simulink model "Copy_of_modelo_completo_sin_joystick"  (R2021a)
settings: Solver=FixedStepAuto  StartTime=0.0  StopTime=inf  FixedStep=0.001  MaxStep=1e-4  RelTol=1e-3
undefined symbols (not defined in the file): bah, bat, bcx, bcy, beqhd, beqt, bw, C_HEIGHT, cols_centers, cols_height, cont_mass, ddxmax, ddxmin, ddymax, ddymin, g, Kcy, Ksah, Ksat, Ksiah, Ksiat, Kw, lh0, Meqh, Meqt, mt, Rd, rt, rth, Rw, sigbuilder_block, sp_mass, VH_MAX, VT_MAX, w_mt_h, w_mt_i, xmax, xt0, ymax, yt0
libraries: simulink x1
(part 2 of 2)

== stateflow chart Copy_of_modelo_completo_sin_joystick/Control Level 1 - Global Supervisor Control1 ==
  state LEVEL1
    entry:
    heights = cols_height;
    centers = cols_centers;
    p0=[0,0];p1=[0,0];p2=[0,0];p3=[0,0];p4=[0,0];p5=[0,0];p6=[0,0];p7=[0,0];p12=[0,0];p23=[0,0];p34=[0,0];p45=[0,0];p56=[0,0];
    [p0,p1,p2,p3,p4,p5,p6,p7,p12,p23,p34,p45,p56] = generate_trajectory(ml,VH_MAX,VT_MAX,heights,centers,single_cycle,double_cycle);
    state MOVEMENT [parallel]
      settings: executionOrder=2
      state AUTOMATIC
        state TO_SHIP
          state HOISTING_ONLY
            state INIT
            state UP
              dxt = 0;
              dlh = -VH_MAX;
            state DOWN
              dxt = 0;
              dlh = VH_MAX;
            (default) -> LEVEL1.MOVEMENT.AUTOMATIC.TO_SHIP.HOISTING_ONLY.INIT
            LEVEL1.MOVEMENT.AUTOMATIC.TO_SHIP.HOISTING_ONLY.INIT -> LEVEL1.MOVEMENT.AUTOMATIC.TO_SHIP.HOISTING_ONLY.DOWN [order 1] : [current_stage==5 && prev_stage==4]
            LEVEL1.MOVEMENT.AUTOMATIC.TO_SHIP.HOISTING_ONLY.INIT -> LEVEL1.MOVEMENT.AUTOMATIC.TO_SHIP.HOISTING_ONLY.UP [order 2] : [current_stage==1&& prev_stage==0]
          state INIT
          state HOISTING_AND_TROLLEY
            state UP
              dxt = VT_MAX;
              dlh = -VH_MAX;
            state DOWN
              dxt = VT_MAX;
              dlh = VH_MAX;
            state INIT
            (default) -> LEVEL1.MOVEMENT.AUTOMATIC.TO_SHIP.HOISTING_AND_TROLLEY.INIT
            LEVEL1.MOVEMENT.AUTOMATIC.TO_SHIP.HOISTING_AND_TROLLEY.INIT -> LEVEL1.MOVEMENT.AUTOMATIC.TO_SHIP.HOISTING_AND_TROLLEY.UP [order 1] : [current_stage == 2 && prev_stage == 1]
            LEVEL1.MOVEMENT.AUTOMATIC.TO_SHIP.HOISTING_AND_TROLLEY.INIT -> LEVEL1.MOVEMENT.AUTOMATIC.TO_SHIP.HOISTING_AND_TROLLEY.DOWN [order 2] : [current_stage== 4 && prev_stage == 3]
          state TROLLEY_ONLY
            dxt = VT_MAX
            dlh = 0;
          (default) -> LEVEL1.MOVEMENT.AUTOMATIC.TO_SHIP.INIT
          LEVEL1.MOVEMENT.AUTOMATIC.TO_SHIP.INIT -> LEVEL1.MOVEMENT.AUTOMATIC.TO_SHIP.HOISTING_ONLY
          LEVEL1.MOVEMENT.AUTOMATIC.TO_SHIP.HOISTING_ONLY -> LEVEL1.MOVEMENT.AUTOMATIC.TO_SHIP.HOISTING_AND_TROLLEY : [current_stage==2 && prev_stage==1]
          LEVEL1.MOVEMENT.AUTOMATIC.TO_SHIP.HOISTING_AND_TROLLEY -> LEVEL1.MOVEMENT.AUTOMATIC.TO_SHIP.HOISTING_ONLY [order 2] : [current_stage == 5 && prev_stage == 4]
          LEVEL1.MOVEMENT.AUTOMATIC.TO_SHIP.HOISTING_AND_TROLLEY -> LEVEL1.MOVEMENT.AUTOMATIC.TO_SHIP.TROLLEY_ONLY [order 1] : [current_stage==3 && prev_stage==2]
          LEVEL1.MOVEMENT.AUTOMATIC.TO_SHIP.TROLLEY_ONLY -> LEVEL1.MOVEMENT.AUTOMATIC.TO_SHIP.HOISTING_AND_TROLLEY : [current_stage == 4 && prev_stage == 3]
        state INIT
        state TO_DOCK
          state HOISTING_ONLY
            state UP
              dxt = 0;
              dlh = -VH_MAX;
            state INIT
            state DOWN
              dxt = 0;
              dlh = VH_MAX;
            (default) -> LEVEL1.MOVEMENT.AUTOMATIC.TO_DOCK.HOISTING_ONLY.INIT
            LEVEL1.MOVEMENT.AUTOMATIC.TO_DOCK.HOISTING_ONLY.INIT -> LEVEL1.MOVEMENT.AUTOMATIC.TO_DOCK.HOISTING_ONLY.UP [order 1] : [current_stage == 5 && prev_stage == 6]
            LEVEL1.MOVEMENT.AUTOMATIC.TO_DOCK.HOISTING_ONLY.INIT -> LEVEL1.MOVEMENT.AUTOMATIC.TO_DOCK.HOISTING_ONLY.DOWN [order 2] : [current_stage == 1&& prev_stage == 2]
          state INIT
          state HOISTING_AND_TROLLEY
            state UP
              dxt = -VT_MAX;
              dlh = -VH_MAX;
            state INIT
            state DOWN
              dxt = -VT_MAX;
              dlh = VH_MAX;
            (default) -> LEVEL1.MOVEMENT.AUTOMATIC.TO_DOCK.HOISTING_AND_TROLLEY.INIT
            LEVEL1.MOVEMENT.AUTOMATIC.TO_DOCK.HOISTING_AND_TROLLEY.INIT -> LEVEL1.MOVEMENT.AUTOMATIC.TO_DOCK.HOISTING_AND_TROLLEY.UP [order 2] : [current_stage == 5 && prev_stage == 6]
            LEVEL1.MOVEMENT.AUTOMATIC.TO_DOCK.HOISTING_AND_TROLLEY.INIT -> LEVEL1.MOVEMENT.AUTOMATIC.TO_DOCK.HOISTING_AND_TROLLEY.DOWN [order 1] : [current_stage == 3 && prev_stage == 4 ]
          state TROLLEY_ONLY
            during:
            dxt = -VT_MAX;
            dlh = 0;
          (default) -> LEVEL1.MOVEMENT.AUTOMATIC.TO_DOCK.INIT
          LEVEL1.MOVEMENT.AUTOMATIC.TO_DOCK.INIT -> LEVEL1.MOVEMENT.AUTOMATIC.TO_DOCK.HOISTING_ONLY
          LEVEL1.MOVEMENT.AUTOMATIC.TO_DOCK.HOISTING_ONLY -> LEVEL1.MOVEMENT.AUTOMATIC.TO_DOCK.HOISTING_AND_TROLLEY : [current_stage == 4 && prev_stage == 5]
          LEVEL1.MOVEMENT.AUTOMATIC.TO_DOCK.HOISTING_AND_TROLLEY -> LEVEL1.MOVEMENT.AUTOMATIC.TO_DOCK.HOISTING_ONLY [order 1] : [current_stage == 1 && prev_stage == 2]
          LEVEL1.MOVEMENT.AUTOMATIC.TO_DOCK.HOISTING_AND_TROLLEY -> LEVEL1.MOVEMENT.AUTOMATIC.TO_DOCK.TROLLEY_ONLY [order 2] : [current_stage == 3 && prev_stage == 4]
          LEVEL1.MOVEMENT.AUTOMATIC.TO_DOCK.TROLLEY_ONLY -> LEVEL1.MOVEMENT.AUTOMATIC.TO_DOCK.HOISTING_AND_TROLLEY : [current_stage == 2 && prev_stage == 3]
        LEVEL1.MOVEMENT.AUTOMATIC.INIT -> TO_SHIP [order 1] : [current_stage == 1 && prev_stage == 0]
        (default) -> LEVEL1.MOVEMENT.AUTOMATIC.INIT
        LEVEL1.MOVEMENT.AUTOMATIC.INIT -> TO_DOCK [order 2] : [current_stage == 5 && prev_stage == 6]
      state MANUAL
        state HYBRID_MANUAL
          state TROLLEY [parallel]
            settings: executionOrder=2
            state STOP
              entry:
              dxt=0;
            state MOVE
              during:
              dxt=VT_MAX*joy_t;
            (default) -> LEVEL1.MOVEMENT.MANUAL.HYBRID_MANUAL.TROLLEY.MOVE
            LEVEL1.MOVEMENT.MANUAL.HYBRID_MANUAL.TROLLEY.STOP -> LEVEL1.MOVEMENT.MANUAL.HYBRID_MANUAL.TROLLEY.MOVE : [joy_t~=0]
            LEVEL1.MOVEMENT.MANUAL.HYBRID_MANUAL.TROLLEY.MOVE -> LEVEL1.MOVEMENT.MANUAL.HYBRID_MANUAL.TROLLEY.STOP : [joy_t==0 || fdct_pos || fdct_neg]
          state HOISTING [parallel]
            settings: executionOrder=1
            state MOVE
              during:
              dlh=VH_MAX*joy_h;
            state STOP
              entry:
              dlh=0;
            (default) -> LEVEL1.MOVEMENT.MANUAL.HYBRID_MANUAL.HOISTING.MOVE
            LEVEL1.MOVEMENT.MANUAL.HYBRID_MANUAL.HOISTING.STOP -> LEVEL1.MOVEMENT.MANUAL.HYBRID_MANUAL.HOISTING.MOVE : [joy_h~=0]
            LEVEL1.MOVEMENT.MANUAL.HYBRID_MANUAL.HOISTING.MOVE -> LEVEL1.MOVEMENT.MANUAL.HYBRID_MANUAL.HOISTING.STOP : [joy_h==0 || fdch_pos || fdch_neg]
        (default) -> HYBRID_MANUAL
      TO_SHIP -> HYBRID_MANUAL : [current_stage == 6 && prev_stage == 5]
      (default) -> MANUAL
      HYBRID_MANUAL -> AUTOMATIC [order 1] : [(current_stage ==  1 && prev_stage == 0) && auto_mode == 1 && ( single_cycle==1 || (double_cycle==1 && charge==1))]
      HYBRID_MANUAL -> AUTOMATIC [order 2] : [current_stage == 5 && prev_stage == 6 && auto_mode == 1 && ( single_cycle==1 || (double_cycle==1 && charge==1)) ]
      TO_DOCK -> HYBRID_MANUAL : [current_stage == 1 && prev_stage == 2]
      AUTOMATIC -> MANUAL : [(joy_t~=0 || joy_h~=0) && auto_mode==0]
    state TRAJECTORY [parallel]
      settings: executionOrder=1
      state STAGE_7
        during:
        current_stage=7;
        exit:
        prev_stage=7;
      state INIT
      state STAGE_0
        during:
        current_stage = 0;
        exit:
        prev_stage=0;
      state STAGE_6
        during:
        current_stage=6;
        exit:
        prev_stage=6;
      state STAGE_1
        during:
        current_stage = 1;
        exit:
        prev_stage=1;
      state STAGE_2
        during:
        current_stage = 2;
        exit:
        prev_stage=2;
      state STAGE_5
        during:
        current_stage=5;
        exit:
        prev_stage=5;
      state STAGE_4
        during:
        current_stage=4;
        exit:
        prev_stage=4;
      state STAGE_3
        during:
        current_stage=3;
        exit:
        prev_stage=3;
      (default) -> LEVEL1.TRAJECTORY.INIT
      LEVEL1.TRAJECTORY.INIT -> STAGE_7 [order 2] : [y>=p7(2)&&x>=p7(1)]
      LEVEL1.TRAJECTORY.INIT -> STAGE_0 [order 1] : [(y>=p0(2) && x>=p0(1))]
      STAGE_0 -> STAGE_1 : [(y>=p1(2) && x>=p1(1))]
      STAGE_1 -> STAGE_0 [order 1] : [(y<=p0(2) && x<=p0(1))]
      STAGE_7 -> STAGE_6 : [y>=p6(2)&&x<=p6(1)]
      STAGE_6 -> STAGE_7 [order 2] : [(y<=p7(2)&&x>=p7(1))]
      STAGE_1 -> STAGE_2 [order 2] : [(y>=p12(2) && x>=p12(1))]
      STAGE_2 -> STAGE_1 [order 2] : [(y<=p1(2)&&x<=p1(1))]
      STAGE_6 -> STAGE_5 [order 1] : [(y>=p5(2)&&x>=p5(1))]
      STAGE_5 -> STAGE_6 [order 2] : [y<=p56(2)]
      STAGE_2 -> STAGE_3 [order 1] : [(y>=p23(2)&&x>=p23(1))]
      STAGE_3 -> STAGE_2 [order 1] : [(y<=p2(2)&&x<=p2(1))]
      STAGE_5 -> STAGE_4 [order 1] : [(y>=p4(2)&&x<=p4(1))]
      STAGE_4 -> STAGE_5 [order 1] : [(y<=p45(2)&&x>=p45(1))]
      STAGE_3 -> STAGE_4 [order 2] : [ x>=p34(1)]
      STAGE_4 -> STAGE_3 [order 2] : [(y>=p3(2) && x<=p3(1))]
  note: Descripcion variables:
      | CARRO (TROLLEY):
      | - move_t -> (variable,int) boton para mover el carro en x.
      | - dx -> (variable,double) velocidad actual del carro (variable)
      | - VXt -> velocidad máxima del carro (es una constante, que al multiplicarla por bot_t modifica el valor de la velocidad real de carro.)
      | - limits_t -> (variable,bool) la variable cambia al valor 1 si se alcanzan los limites de movimiento del carro.
      |
      | IZAJE (HOISTING):
      | - move_h ->(variable,int) boton para izar la carga.
      | - dy -> (variable,double) velocidad actual del izaje.
      | - VYh -> (constante) velocidad máxima que puede alcanzar el izaje.
      | - limits_h -> (variable,bool) la variable cambia al valor 1 si se alcanzan los limites de movimiento del izaje.
      |
      | Descripcion de bloques:
      | - ALL_MANUAL:
      | Es el modo manual por defecto, el operario puede manejar el trolley y el hoisting con 2 botones. El boton move_t se encarga de mover el trolley y el boton move_h de izar la carga.
      | - HYRBID_MANUAL:
      | Es el modo manual que esta presente en los ciclos simple o doble. Es decir, esta intercalado con el modo automático
  note: Descripción de ciclos:
      | -SIMPLE:
      | O se carga o se descarga, es decir: Si estoy cargando el barco, en el tramo muelle -> barco llevo un contenedor, pero vuelvo vacio. Es decir que el tramo barco -> muelle es sin ningun contenedor. Lo mismo sucederia si estoy descargando el barco: el tramo barco -> muelle es con un contenedor cargado, pero el tramo muelle -> barco es en vacio.
      | - DOBLE:
      | Se puede cargar y descargar en el mismo ciclo de trabajo. Es decir, que el tramo muelle -> barco es con un contenedor cargado, y el tramo barco -> muelle también. Por ende, se permite una carga intermedia antes de volver al muelle.
      |
      | ETAPAS DE LA TRAYECTORIA:
      | Cada stage se va aactivando dependiendo del punto de la trayectoria en el que se encuentra el barco
      | - STAGE 1 -> ground - el contenedor esta en tierra
      | - STAGE 2 -> el contenedor se encuentra en el aire (sobre muelle), en el punto de transicion manual a automatico.
      | - STAGE 3 -> el contenedor se enceuntra en el aire (sobre barco) ,en el punto de transicion automatico a manual.
      | - STAGE 4 -> el contenedor se encuentra en el barco.
  data: ml_ function_input; VH_MAX_ function_input; VT_MAX_ function_input; cols_height_ function_input; cols_centers_ function_input; single_cycle_ function_input; double_cycle_ function_input; p00 function_output; p11 function_output; p22 function_output; p33 function_output; p44 function_output; p55 function_output; p66 function_output; p77 function_output; p1122 function_output; p2233 function_output; p3344 function_output; p4455 function_output; p5566 function_output; fdct_pos input; fdct_neg input; fdch_pos input; fdch_neg input; dxt output; dlh output; y input; joy_t input; joy_h input; auto_mode input; x input; prev_stage local =0; current_stage local =0; single_cycle input; double_cycle input; VH_MAX input; VT_MAX input; charge input; p0 local; p1 local; p2 local; p3 local; p4 local; p5 local; p6 local; p7 local; cols_centers input; cols_height input; heights local; centers local; ml input; p12 local; p23 local; p34 local; p45 local; p56 local
  function [p00,p11,p22,p33,p44,p55,p66,p77,p1122,p2233,p3344,p4455,p5566]      = generate_trajectory (ml_,VH_MAX_,VT_MAX_, cols_height_,cols_centers_,single_cycle_,double_cycle_):
    | function [p00,p11,p22,p33,p44,p55,p66,p77,p1122,p2233,p3344,p4455,p5566]      = generate_trajectory (ml_,VH_MAX_,VT_MAX_, cols_height_,cols_centers_,single_cycle_,double_cycle_)
    | 
    | weight = ml_;
    | to_where = 'to_ship';
    | plt_traj = "true";
    | cycle_type = "single";
    | 
    | %% Defincion de los parametros iniciales previo a comenzar el trayecto
    | 
    | if single_cycle_ == 1
    |     cycle_type = "single";
    | else
    |     if double_cycle_ == 1
    |         cycle_type = "double";
    |     end
    | end
    | 
    | % Definimos dimensiones de un contendor maritimo [metros]
    | C_HEIGHT = 2.89;
    | C_WIDTH = 2.438;
    | c_weight = weight;
    | 
    | % Definimos dimensiones del barco (ship) [metros]
    | N_COLS = 9; % Cantidad de columnas del barco
    | MAX_C_OVER_DOCK= 9; % Cantidad maxima de containers sobre nivel del muelle
    | 
    | %% Comienzo de generacion de la trayectoria dependiendo de la situacion
    | slope=atan(VH_MAX_/VT_MAX_); %pendiente
    | 
    | % Definimos el punto de inicio (p1) en el muelle con coordenadas x,y
    | p0=[-20,0];
    | 
    | % Generamos un numero aleatorio que nos dice a que numero de columna debemos llevar el contenedor. Definimos asi p6.
    | while(1)
    |     %index_goal=randi([1,N_COLS],1,1);
    |     index_goal = 9;
    |     if cols_height_(index_goal)<C_HEIGHT*MAX_C_OVER_DOCK
    |         break;
    |     end
    | end
    | %index_goal=1;
    | p7=[cols_centers_(index_goal),cols_height_(index_goal)];
    | 
    | % Generamos un vector que solo contenga las columnas a la izquierda del punto objetivo. Son los unicos puntos que importan.
    | left_cols=cols_height_(1:index_goal);
    | 
    | % Buscamos los de las columnas de mayor altura , tanto la que se encuentra mas a la izquierda como la que se encuentra mas a la
    | % derecha.
    | max=0;
    | imax_left=0;
    | imax_right=0;
    | for i=1:index_goal
    |     if left_cols(i)>=max
    |         imax_right=i;
    |         if left_cols(i)>max
    |             imax_left=i;
    |         end
    |     max=left_cols(i);
    |     end
    | end
    | 
    | %% Calculo de p3 y p2
    | 
    | % Definimos la altura de seguridad que me definira la coord y de p3.
    | % Se considera la altura de 2 contenedores para seguridad
    | H_SAFE=max+2*C_HEIGHT;
    | 
    | % Definimos el x de seguridad, que define la coord. x de p3
    | % Se considera el ancho de un contenedor para seguridad
    | x_safe=cols_centers_(imax_left)-C_WIDTH;
    | 
    | % Primer valor de p3, sin verificacion aun.
    | p3=[x_safe,H_SAFE];
    | 
    | % Definimos p2 usando trigonometria.
    | p2=[-20, p3(2)-tan(slope)*(p3(1)-p0(1))];
    | 
    | % Bucle que verifica que la trayectoria de p3 a p2 no con otra columna. Si esto ocurre, modificamos el valor de p3
    | % y por ende de p2.
    | e=0;
    | next_index=imax_left-1;
    | while next_index>0
    | 
    |    % y23 indica el valor de la recta que une p2 con p3 en el punto
    |    % central de cada columna.
    |    y23=p3(2)-tan(slope)*(p3(1)-cols_centers_(next_index));
    | 
    |    % Verificamos que no haya colision entre la recta que une p2
    |    % con p3 (mas una distancia de seguridad) y la columna.
    |    if y23<cols_height_(next_index)+2*C_HEIGHT
    | 
    |         % Si hay colision, entonces debemos actualizar p3 y por
    |         % ende, p2. Para actualizar p3 se corre un ancho a la
    |         % izquierda el punto x de p3.
    |         e=e+1;
    |         p3=[x_safe-e*C_WIDTH,H_SAFE];
    |         p2=[-20, p3(2)-tan(slope)*(p3(1)-p0(1))];
    |         next_index=imax_left;
    |    end
    |    next_index=next_index-1;
    | end
    | 
    | 
    | %%  Calculo de p4 y p5
    | 
    | % Si el contenedor tiene que ir a la primer columna, o tiene que ir
    | % a un maximo el p4 y p5 en x seran igual al p6 x. En altura seran
    | %la altura de seguridad
    | if (index_goal ==1 || max==left_cols(index_goal))
    |     p4=[p7(1),H_SAFE];
    |     p5=p4;
    | 
    | else
    |     % Definimos el x de seguridad, que define la coord. x de p3
    |     % Se considera el ancho de un contenedor para seguridad
    |     x_safe=cols_centers_(imax_right)+C_WIDTH;
    | 
    |     % Primer valor de p4, sin verificacion aun.
    |     p4=[x_safe,H_SAFE];
    | 
    |     % Definimos p5 usando trigonometria.
    |     p5=[p7(1), p4(2)+tan(slope)*(p4(1)-p7(1))];
    |     % Bucle que verifica que la trayectoria de p4 a p5 no con otra
    |     % columna. Si esto ocurre, modificamos el valor de p4
    |     % y por ende de p5.
    |     e=0;
    |     next_index=imax_right+1;
    |     while next_index<=index_goal
    | 
    |        % y45 indica el valor de la recta que une p4 con p5 en el punto
    |        % central de cada columna.
    |        y45=p4(2)+tan(slope)*(p4(1)-cols_centers_(next_index));
    | 
    |        % Verificamos que no haya colision entre la recta que une p4
    |        % con p5 (mas una distancia de seguridad) y la columna.
    |        if y45<cols_height_(next_index)+2*C_HEIGHT
    | 
    |             % Si hay colision, entonces debemos actualizar p4 y por
    |             % ende, p5. Para actualizar p4 se corre un ancho a la
    |             % derecha el punto x de p4.
    |             e=e+1;
    |             p4=[x_safe+e*C_WIDTH,H_SAFE];
    |             p5=[p7(1), p4(2)+tan(slope)*(p4(1)-p7(1))];
    |             next_index=imax_right;
    |        end
    |        next_index=next_index+1;
    |     end
    | end
    | 
    | p1 = [p0(1),(p2(2)-p0(2))/2];
    | p6 = [p7(1),(p5(2)-p7(2))/2+p7(2)];
    | 
    | switch(to_where)    
    |     case 'to_ship' 
    |     % En este caso los puntos seran como se calcularon.
    |       
    |     case 'to_dock'       
    |     % En este caso se invierten los puntos, el p1 sera aleatorio y el p6
    |     % será un punto fijo en (-20,0). Primero guardamos los puntos en puntos
    |     % auxiliares y luego se actualizan.
    |     p0d=p0;
    |     p1d=p1;
    |     p2d=p2;
    |     p3d=p3;
    |     p4d=p4;
    |     p5d=p5;
    |     p6d=p6;
    |     p7d=p7;
    |     p7=p7d;
    |     p6=p1d;
    |     p5=p2d;
    |     p4=p3d;
    |     p3=p4d;
    |     p2=p5d;
    |     p1=p6d;
    |     p0=p0d;
    |    
    | end % end switch
    | 
    | p00 = p0;
    | p11 = p1;
    | p22 = p2;
    | p33 = p3;
    | p44 = p4;
    | p55 = p5;
    | p66 = p6;
    | p77 = p7;
    | 
    | %% Definimos puntos guia cuando falte el 10% para llegar al siguiente punto
    | % para que en ese punto comience a bajar la velocidad de a poco
    | route_percent_1 = 0.80;
    | route_percent_2 = 0.60;
    | p1122 = [p1(1) + (p2(1) - p1(1))*route_percent_1,p1(2) + (p2(2) - p1(2))*route_percent_1];
    | p2233 = [p2(1) + (p3(1) - p2(1))*route_percent_1,p2(2) + (p3(2) - p2(2))*route_percent_1];
    | p3344 = [p3(1) + (p4(1) - p3(1))*route_percent_2,p3(2) + (p4(2) - p3(2))*route_percent_2];
    | p4455 = [p4(1) + (p5(1) - p4(1))*route_percent_2,p4(2) + (p5(2) - p4(2))*route_percent_2];
    | p5566 = [p5(1) + (p6(1) - p5(1))*route_percent_1,p5(2) + (p6(2) - p5(2))*route_percent_1];
    | 
    | end % end function

== matlab function Copy_of_modelo_completo_sin_joystick/Level 2 control + Physical model1/Control Level 2/PD of load balance /Ganancias control theta ==
  data: mt input; ml input; Kp output; Kd output; Meqt input; lh input
function [Kp,Kd] = PD_balanceo(mt, ml, Meqt,lh)
%G = tf([-(mt+ml) 0],[(Meqt+ml)*lh 0 Meqt]);
g=9.81;
mod = abs(sqrt(complex(-(Meqt*g)/((Meqt+ml)*lh))));
w_pos = mod*10;
mEq = -(Meqt+ml)*lh/(mt+ml);
nb = 3;
Kd = mEq*nb*w_pos;
Kp = mEq*nb*(w_pos^2);
%Kd=(-((Meqt*g)/(w_pos^2))+((Meqt+ml)*lh))/(ml+mt);
%Kp=2*w_pos*(-lh*((Meqt+ml)/(ml+mt))+Kd);

end

== matlab function Copy_of_modelo_completo_sin_joystick/Level 2 control + Physical model1/Physical model/get_obstacles_profile ==
  data: xl input; yc0xt output; cols_centers input; cols_height input; ml input; xmax input
function yc0xt = getYc0x(xl,cols_centers,cols_height, ml,xmax)
%{
@type MATLAB function called from SIMULINK
@name get_obstacles_profile
@description - Obtiene el perfil de obstaculos 
@params {float,simulation} xl - valor en tiempo real de la posocion del
carro
@params {array} cols_centers - Contiene las coordenadas de los centros de
cada columna. Array de 1xN , con N = cantidad de columnas
@params {cols_heights} - Altura de cada columna respecto del punto 0,0.
@returns {float} yc0xt - Valor en altura del obstaculo para la coordenada
xl, en el instante de tiempo t actual.
%}

yc0xt = 2.6;
aux = 0;
indice = 1;
C_WIDTH = 2.5;
if(xl <= 0)
    yc0xt = 0;
    
elseif (xl >= xmax)
    yc0xt = 0;
    
elseif (xl > 0)
   for i=1:length(cols_centers)
       % xl hasta centro columna
       x_comp = xl-cols_centers(i);
        if(x_comp>= -C_WIDTH && x_comp<0)
            if (i ~= 1 && cols_height(i-1)>=cols_height(i))
                indice = i-1;
            else
                indice = i;
            end
        elseif(x_comp == 0)
            indice = i;
        elseif(x_comp<= C_WIDTH && x_comp>0)
            if (i ~= length(cols_centers) && cols_height(i+1)>=cols_height(i))
                indice = i+1;
            else
                indice = i;
            end
        end 
    end
    yc0xt=cols_height(indice);
end

if(ml > 17000) % Si el spreader esta cargado
    yc0xt = yc0xt + C_WIDTH/2;
end


end %end function
